simulink model "outmod_mdl"  (R2021b)
settings: Solver=ode1  StartTime=0.0  StopTime=150  FixedStep=0.0001  MaxStep=0.1  MinStep=0.01  RelTol=1e-3
values from neighbouring files (symbols this model uses):
  A = [0 1; 0 0]    [pendulum_data.m]
  Am = A+B*Lx    [obsmod_data.m]    (also in outmod_data.m; outmodc_data.m; stmod_data.m = A+B*F)
  B = [0;1]    [pendulum_data.m]
  Bm = B*-inv(Cm*inv(Am)*B)    [obsmod_data.m]    (also in outmod_data.m; outmodc_data.m; stmod_data.m = B*G)
  C = C([1,3],:)    [comp_data.m]    (also in pendulum_data.m = [1 1])
  gammac = -1.5*eye(m)    [outmod_data.m]
  rho = 1    [comp_data.m]    (also in obsint_data.m; obsmod_data.m; outmod_data.m; outmodc_data.m)
  x0 = zeros(1,n)    [comp_data.m]    (also in obsint_data.m; obsmod_data.m; outmod_data.m; outmodc_data.m)
undefined symbols (not defined in the file or in its folder): Cm, F, Lr, Lx, m, n, p
settings Model: Creator=w.schwamm  LastModifiedBy=Witali
settings DataIOCC: SaveOutput=off  SaveTime=off  ReturnWorkspaceOutputs=off  StateSaveName=x  TimeSaveName=t  OutputSaveName=y

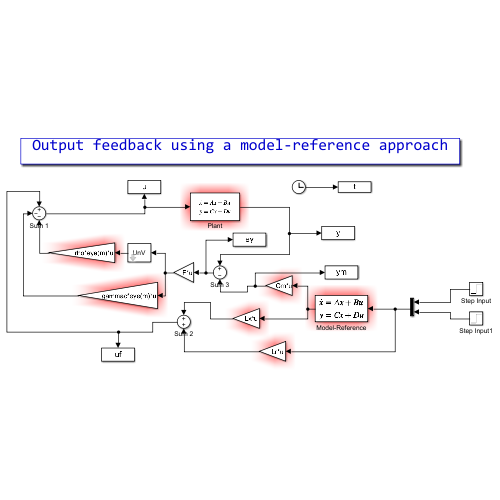
[thumbnail: Simulink's stored preview of the top-level diagram]
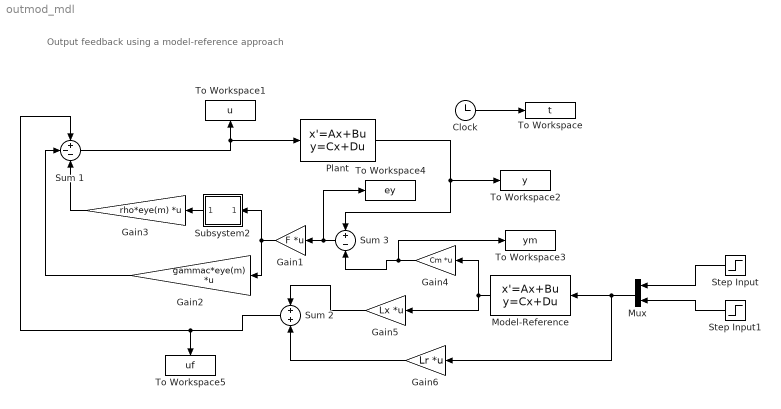
== system outmod_mdl ==
  note: Output feedback using a model-reference approach
  Clock : Clock
  Gain1 : Gain  Gain=F  Multiplication=Matrix(K*u)
  Gain2 : Gain  Gain=gammac*eye(m)  Multiplication=Matrix(K*u)
  Gain3 : Gain  Gain=rho*eye(m)  Multiplication=Matrix(K*u)
  Gain4 : Gain  Gain=Cm  Multiplication=Matrix(K*u)
  Gain5 : Gain  Gain=Lx  Multiplication=Matrix(K*u)
  Gain6 : Gain  Gain=Lr  Multiplication=Matrix(K*u)
  Model-Reference : StateSpace  A=Am  B=Bm  C=eye(n)  D=zeros(n,m)  InitialCondition=0
  Mux : Mux  Inputs=2
  Plant : StateSpace  A=A  B=B  C=C  D=zeros(p,m)  InitialCondition=x0
  Step Input : Step  Time=0  SampleTime=0
  Step Input1 : Step  Time=0  After=0  SampleTime=0
  Subsystem2 : Subsystem  mask{delta=0.01}
      mask prompts: delta "Unit vector delta:"
      mask Display: disp('UnV')
  Sum 1 : Sum  Inputs=+--
  Sum 2 : Sum
  Sum 3 : Sum  Inputs=+-
  To Workspace : ToWorkspace  VariableName=t  SaveFormat=Timeseries  SampleTime=-1
      settings: MaxDataPoints=1000000
  To Workspace1 : ToWorkspace  VariableName=u  SaveFormat=Timeseries  SampleTime=-1
      settings: MaxDataPoints=1000000
  To Workspace2 : ToWorkspace  VariableName=y  SaveFormat=Timeseries  SampleTime=-1
      settings: MaxDataPoints=1000000
  To Workspace3 : ToWorkspace  VariableName=ym  SaveFormat=Timeseries  SampleTime=-1
      settings: MaxDataPoints=1000000
  To Workspace4 : ToWorkspace  VariableName=ey  SaveFormat=Timeseries  SampleTime=-1
      settings: MaxDataPoints=1000000
  To Workspace5 : ToWorkspace  VariableName=uf  SaveFormat=Timeseries  SampleTime=-1
      settings: MaxDataPoints=1000000
  wires:
  Model-Reference/1 -> Gain5/1, Gain4/1
  Plant/1 -> To Workspace2/1, Sum 3/1
  Subsystem2/1(Out1) -> Gain3/1
  Sum 3/1 -> Gain1/1, To Workspace4/1
  Gain3/1 -> Sum 1/3
  Gain2/1 -> Sum 1/2
  Gain5/1 -> Sum 2/1
  Gain6/1 -> Sum 2/2
  Sum 2/1 -> Sum 1/1, To Workspace5/1
  Clock/1 -> To Workspace/1
  Sum 1/1 -> Plant/1, To Workspace1/1
  Gain4/1 -> Sum 3/2, To Workspace3/1
  Step Input1/1 -> Mux/2
  Mux/1 -> Gain6/1, Model-Reference/1
  Step Input/1 -> Mux/1
  Gain1/1 -> Subsystem2/1(In1), Gain2/1

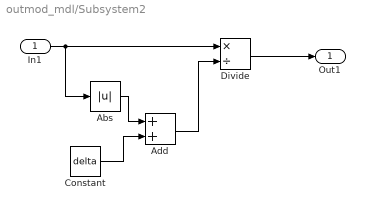
== system outmod_mdl/Subsystem2 ==
  In1 : Inport
  Abs : Abs
  Add : Sum
  Constant : Constant  Value=delta  SampleTime=-1
  Divide : Product  Inputs=*/
  Out1 : Outport
  wires:
  Constant/1 -> Add/2
  Add/1 -> Divide/2
  Abs/1 -> Add/1
  Divide/1 -> Out1/1
  In1/1 -> Divide/1, Abs/1
